simulink model "sim_example_2_1"  (R2020b)
settings: Solver=ode45  StartTime=0.0  StopTime=10.0  RelTol=1e-3  EnableMultiTasking=on
libraries: simulink x1
settings Model: Creator=Ahmadieh  LastModifiedBy=mojta
settings DataIOCC: LimitDataPoints=on  SaveFormat=Array  ReturnWorkspaceOutputs=off
settings OptimizationCC: LifeSpan=inf
settings DebuggingCC: UnderspecifiedInitializationDetection=Classic  MergeDetectMultiDrivingBlocksExec=none  SolverPrmCheckMsg=warning  SFUnexpectedBacktrackingDiag=warning  SFNoUnconditionalDefaultTransitionDiag=warning  SFExecutionAtInitializationDiag=none  ArithmeticOperatorsInVariantConditions=warning
settings HardwareCC: ProdBitPerPointer=32  ProdBitPerSizeT=32  ProdBitPerPtrDiffT=32  ProdLargestAtomicFloat=None  ProdIntDivRoundTo=Undefined  ProdEndianess=Unspecified  ProdWordSize=32  ProdHWDeviceType=32-bit Generic
settings ModelReferenceCC: PropagateSignalLabelsOutOfModel=off
settings SFSimCC: SimUseLocalCustomCode=off  CustomCodeUndefinedFunction=UseInterfaceOnly
settings RTWCC: RTWUseLocalCustomCode=off
settings CodeAppCC: StateflowObjectComments=on
settings GRTTargetCC: TargetLangStandard=C89/C90 (ANSI)
settings ConfigComp: CovMetricSettings=dw  CovSaveCumulativeToWorkspaceVar=on  CovSaveSingleToWorkspaceVar=on  CovExternalEMLEnable=off

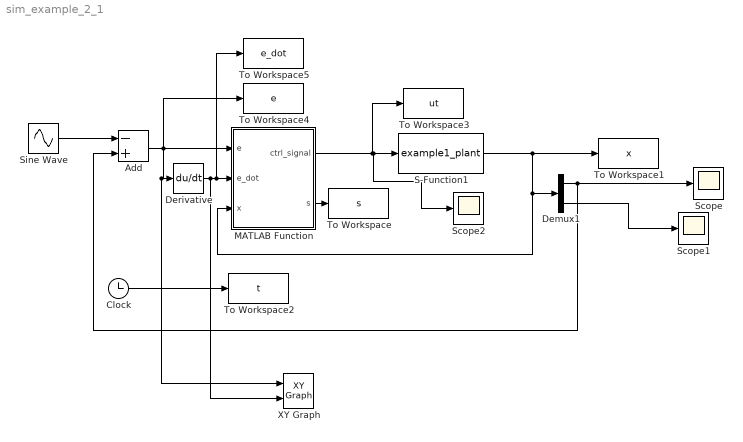
== system sim_example_2_1 ==
  Add : Sum  Inputs=-+
  Clock : Clock
  Demux1 : Demux  Outputs=2
  Derivative : Derivative
  MATLAB Function : MATLAB Function  TreatAsAtomicUnit=on
  S-Function1 : S-Function  FunctionName=example1_plant  SFunctionDeploymentMode=off  EnableBusSupport=off
  Scope : Scope
  Scope1 : Scope
  Scope2 : Scope
  Sine Wave : Sin  SampleTime=0
  To Workspace : ToWorkspace  VariableName=s  SampleTime=-1
  To Workspace1 : ToWorkspace  VariableName=x  SampleTime=-1
  To Workspace2 : ToWorkspace  VariableName=t  SampleTime=-1
  To Workspace3 : ToWorkspace  VariableName=ut  SampleTime=-1
  To Workspace4 : ToWorkspace  VariableName=e  SampleTime=-1
  To Workspace5 : ToWorkspace  VariableName=e_dot  SampleTime=-1
  XY Graph : simulink/Sinks/XY Graph  xmin=-1  xmax=1  ymin=-1  ymax=1  st=-1
  wires:
  S-Function1/1 -> To Workspace1/1, Demux1/1, MATLAB Function/3(x)
  Clock/1 -> To Workspace2/1
  Add/1 -> To Workspace4/1, XY Graph/1, Derivative/1, MATLAB Function/1(e)
  Sine Wave/1 -> Add/1
  Demux1/1 -> Add/2, Scope/1
  Derivative/1 -> MATLAB Function/2(e_dot), To Workspace5/1, XY Graph/2
  MATLAB Function/1(ctrl_signal) -> To Workspace3/1, Scope2/1, S-Function1/1
  MATLAB Function/2(s) -> To Workspace/1
  Demux1/2 -> Scope1/1

== matlab function sim_example_2_1/MATLAB Function ==
  data: e input; ctrl_signal output; e_dot input; s output; x input
function [ctrl_signal,s] = fcn(e,e_dot,x)
%#codegen
s=e+e_dot;
g=9.8;mc=1.0;m=0.1;l=1;a=1/(mc+m);
x1=x(1);
x2=x(2);
ctrl_signal=(-g*sin(x1)+m*l*a^2*x2^2*cos(x1)*sin(x1)-3*sat(s,0.1))/l/...
    (a*cos(x1));
end

function y=sat(s,eps)
if abs(s)<eps
    y=s/eps;
else
    y=sign(s);
end
end
